simulink model "Attitude_Determination_Iterated"  (R2016b)
settings: Solver=FixedStepDiscrete  StartTime=0.0  StopTime=1  FixedStep=0.1  RelTol=1e-3
undefined symbols (not defined in the file or in its folder): km, s
libraries: dspmathops x4, aerolibtransform2 x1, aerolibgravity2 x1, aerolibcelestial x1
settings Model: Creator=Patipan  LastModifiedBy=Patipan

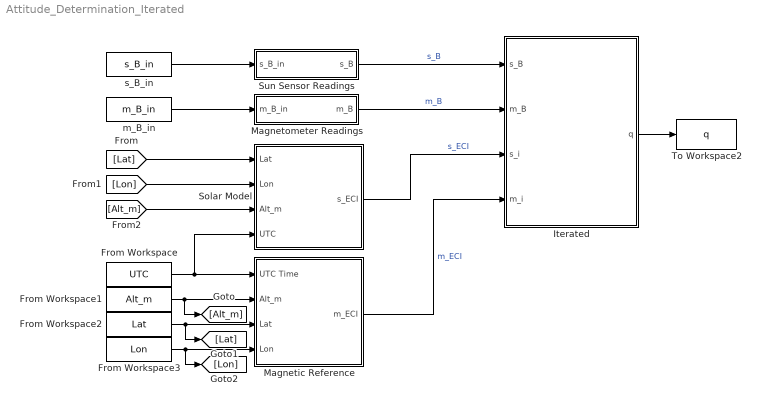
== system Attitude_Determination_Iterated ==
  From Workspace : FromWorkspace  VariableName=UTC  SampleTime=0
  From Workspace1 : FromWorkspace  VariableName=Alt_m  SampleTime=0
  From Workspace2 : FromWorkspace  VariableName=Lat  SampleTime=0
  From Workspace3 : FromWorkspace  VariableName=Lon  SampleTime=0
  Iterated : MATLAB Function  TreatAsAtomicUnit=on
  Magnetic Reference : Subsystem
  Magnetometer Readings : Subsystem
  Solar Model : Subsystem
  Sun Sensor Readings : Subsystem
  To Workspace2 : ToWorkspace  VariableName=q  SampleTime=-1
      settings: Save2DSignal=2-D array (concatenate along first dimension)
  m_B_in : FromWorkspace  VariableName=m_B_in  SampleTime=0
  "s_B_in " : FromWorkspace  VariableName=s_B_in  SampleTime=0
  wires:
  Sun Sensor Readings/1(s_B) -> Iterated/1(s_B)  "s_B"
  Magnetometer Readings/1(m_B) -> Iterated/2(m_B)  "m_B"
  Solar Model/1(s_ECI) -> Iterated/3(s_i)  "s_ECI"
  Magnetic Reference/1(m_ECI) -> Iterated/4(m_i)  "m_ECI"
  "s_B_in "/1 -> Sun Sensor Readings/1(s_B_in)
  m_B_in/1 -> Magnetometer Readings/1(m_B_in)
  From Workspace/1 -> Solar Model/4(UTC), Magnetic Reference/1(UTC Time)
  From Workspace1/1 -> [Alt_m], Magnetic Reference/2(Alt_m)
  From Workspace2/1 -> [Lat], Magnetic Reference/3(Lat)
  From Workspace3/1 -> [Lon], Magnetic Reference/4(Lon)
  [Lat] -> Solar Model/1(Lat)
  [Lon] -> Solar Model/2(Lon)
  [Alt_m] -> Solar Model/3(Alt_m)
  Iterated/1(q) -> To Workspace2/1

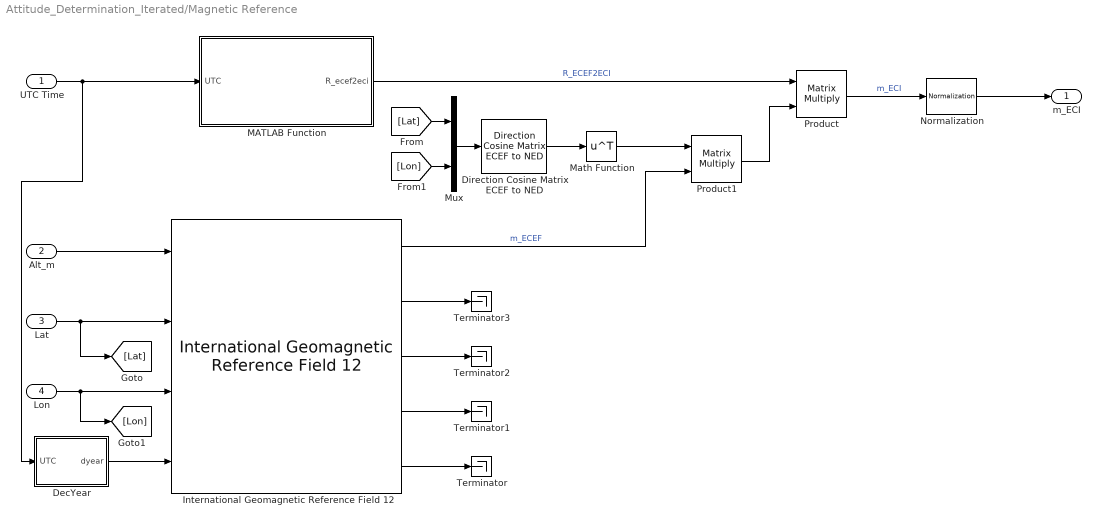
== system Attitude_Determination_Iterated/Magnetic Reference ==
  UTC Time : Inport
  Alt_m : Inport  Port=2
  Lat : Inport  Port=3
  Lon : Inport  Port=4
  DecYear : MATLAB Function  TreatAsAtomicUnit=on
  Direction Cosine Matrix ECEF to NED : aerolibtransform2/Direction Cosine Matrix ECEF to NED
  International Geomagnetic Reference Field 12 : aerolibgravity2/International Geomagnetic Reference Field 12  units=Metric (MKS)  time_in=on  month=January  day=1  year=2020  action=None  sv_out=off
  MATLAB Function : MATLAB Function  TreatAsAtomicUnit=on
  Math Function : Math  Operator=transpose  SaturateOnIntegerOverflow=on
  Mux : Mux  Inputs=2
  Normalization : dspmathops/Normalization  NormType=2-norm  Bias=1e-10  NormOver=Each column  Dimension=1  outputDataTypeStr=Inherit: Same as product output  outputLastDataTypeStr=Inherit: Same as product output  outputMin=[]  outputMax=[]  accumDataTypeStr=Inherit: Same as product output  accumLastDataTypeStr=Inherit: Same as product output  roundingMode=Floor  overflowMode=off
  Product : Product  Multiplication=Matrix(*)
  Product1 : Product  Multiplication=Matrix(*)
  Terminator{,1..3} (4 alike) : Terminator
  m_ECI : Outport
  wires:
  International Geomagnetic Reference Field 12/2 -> Terminator3/1
  International Geomagnetic Reference Field 12/3 -> Terminator2/1
  MATLAB Function/1(R_ecef2eci) -> Product/1  "R_ECEF2ECI"
  Product/1 -> Normalization/1  "m_ECI"
  International Geomagnetic Reference Field 12/4 -> Terminator1/1
  International Geomagnetic Reference Field 12/5 -> Terminator/1
  Lon/1 -> [Lon], International Geomagnetic Reference Field 12/3
  UTC Time/1 -> DecYear/1(UTC), MATLAB Function/1(UTC)
  Alt_m/1 -> International Geomagnetic Reference Field 12/1
  Lat/1 -> [Lat], International Geomagnetic Reference Field 12/2
  DecYear/1(dyear) -> International Geomagnetic Reference Field 12/4
  Mux/1 -> Direction Cosine Matrix ECEF to NED/1
  [Lat] -> Mux/1
  [Lon] -> Mux/2
  International Geomagnetic Reference Field 12/1 -> Product1/2  "m_ECEF"
  Direction Cosine Matrix ECEF to NED/1 -> Math Function/1
  Math Function/1 -> Product1/1
  Product1/1 -> Product/2
  Normalization/1 -> m_ECI/1

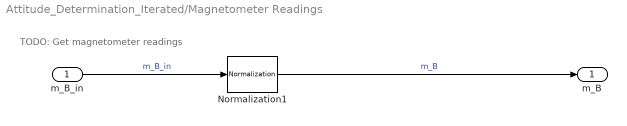
== system Attitude_Determination_Iterated/Magnetometer Readings ==
  note: TODO: Get magnetometer readings
  m_B_in : Inport
  Normalization1 : dspmathops/Normalization  NormType=2-norm  Bias=1e-10  NormOver=Each column  Dimension=1  outputDataTypeStr=Inherit: Same as product output  outputLastDataTypeStr=Inherit: Same as product output  outputMin=[]  outputMax=[]  accumDataTypeStr=Inherit: Same as product output  accumLastDataTypeStr=Inherit: Same as product output  roundingMode=Floor  overflowMode=off
  m_B : Outport
  wires:
  Normalization1/1 -> m_B/1  "m_B"
  m_B_in/1 -> Normalization1/1  "m_B_in"

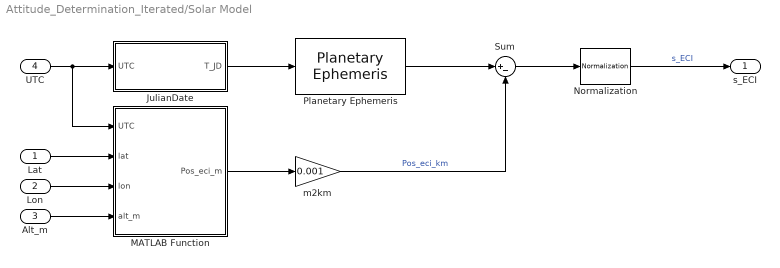
== system Attitude_Determination_Iterated/Solar Model ==
  Lat : Inport
  Lon : Inport  Port=2
  Alt_m : Inport  Port=3
  UTC : Inport  Port=4
  JulianDate : MATLAB Function  TreatAsAtomicUnit=on
  MATLAB Function : MATLAB Function  TreatAsAtomicUnit=on
  Normalization : dspmathops/Normalization  NormType=2-norm  Bias=1e-10  NormOver=Each column  Dimension=1  outputDataTypeStr=Inherit: Same as product output  outputLastDataTypeStr=Inherit: Same as product output  outputMin=[]  outputMax=[]  accumDataTypeStr=Inherit: Same as product output  accumLastDataTypeStr=Inherit: Same as product output  roundingMode=Floor  overflowMode=off
  Planetary Ephemeris : aerolibcelestial/Planetary Ephemeris  kmflag=km,km/s  epochflag=Julian date  de=DE423  nCenter=Earth  nTarget=Sun  errorflag=Error  velflag=off
  Sum : Sum  Inputs=|+-
  m2km : Gain  Gain=0.001
  s_ECI : Outport
  wires:
  Normalization/1 -> s_ECI/1  "s_ECI"
  JulianDate/1(T_JD) -> Planetary Ephemeris/1
  UTC/1 -> MATLAB Function/1(UTC), JulianDate/1(UTC)
  Lat/1 -> MATLAB Function/2(lat)
  Lon/1 -> MATLAB Function/3(lon)
  Alt_m/1 -> MATLAB Function/4(alt_m)
  MATLAB Function/1(Pos_eci_m) -> m2km/1
  Planetary Ephemeris/1 -> Sum/1
  m2km/1 -> Sum/2  "Pos_eci_km"
  Sum/1 -> Normalization/1

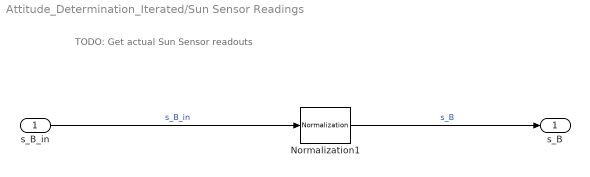
== system Attitude_Determination_Iterated/Sun Sensor Readings ==
  note: TODO: Get actual Sun Sensor readouts
  s_B_in : Inport
  Normalization1 : dspmathops/Normalization  NormType=2-norm  Bias=1e-10  NormOver=Each column  Dimension=1  outputDataTypeStr=Inherit: Same as product output  outputLastDataTypeStr=Inherit: Same as product output  outputMin=[]  outputMax=[]  accumDataTypeStr=Inherit: Same as product output  accumLastDataTypeStr=Inherit: Same as product output  roundingMode=Floor  overflowMode=off
  s_B : Outport
  wires:
  Normalization1/1 -> s_B/1  "s_B"
  s_B_in/1 -> Normalization1/1  "s_B_in"

== matlab function Attitude_Determination_Iterated/Magnetic Reference/MATLAB Function ==
  data: UTC input; R_ecef2eci output
function R_ecef2eci  = ecef2eci(UTC)
% Output rotation matrix from Earth-Centered Earth-Fixed frame to Earth
% Inertial frame from UTC time array.
%  

coder.extrinsic('dcmeci2ecef')

R_eci2ecef = zeros(3, 3);
R_eci2ecef = dcmeci2ecef('IAU-76/FK5', UTC');

R_ecef2eci = R_eci2ecef';
end

== matlab function Attitude_Determination_Iterated/Solar Model/JulianDate ==
  data: UTC input; T_JD output
function T_JD = JulianDate(UTC)

coder.extrinsic('juliandate')
T_JD = 0;
T_JD = juliandate(UTC');

== matlab function Attitude_Determination_Iterated/Magnetic Reference/DecYear ==
  data: UTC input; dyear output
function dyear = DecYear(UTC)

coder.extrinsic('decyear');
dyear = 0;
dyear = decyear(UTC');

== matlab function Attitude_Determination_Iterated/Solar Model/MATLAB Function ==
  data: UTC input; Pos_eci_m output; lat input; lon input; alt_m input
function Pos_eci_m  = lla2eci(UTC, lat, lon, alt_m)
% Output rotation matrix from Earth-Centered Earth-Fixed frame to Earth
% Inertial frame from UTC time array.
%  

coder.extrinsic('lla2eci')

Pos_eci_m = zeros(3, 1);
Pos_eci_m = lla2eci([lat lon alt_m], UTC');

end

== matlab function Attitude_Determination_Iterated/Iterated ==
  data: s_B input; m_B input; s_i input; m_i input; q output
function q  = Iterated(s_B, m_B, s_i, m_i)
% This function is the extended kalman filter for CubeSat attitude
% determination.
% INPUT:
% s_B       Sun vector in body frame from sun sensors
% m_B       Magnetic field vector in body frame from magnetometers
% s_i       Sun vector in inertial frame from planetary ephemeris model
% m_i       Magnetic field vector in inertial frame from IGRF model
%
% OUTPUT:  
% q         Attitude quaternion estimate of the satellite
%

coder.extrinsic('quatrotate');
dt = 0.1; % period for data processing
%% Initialize attitude and error
q = [1 0 0 0];
qprev = [1 0 0 0];
m_est = zeros(3, 1);
s_est = zeros(3, 1);
%% Iterate
for i=1:20
    m_est = quatrotate(q, m_i')';
    s_est = quatrotate(q, s_i')';
    dm = m_B - m_est;
    ds = s_B - s_est;
    
    H = -2*[0               m_est(3)      -m_est(2); 
            -m_est(3)       0             m_est(1);
            m_est(2)        -m_est(1)     0;
            0               s_est(3)      -s_est(2);
            -s_est(3)       0             s_est(1);
            s_est(2)        -s_est(1)     0]; % [6x3] matrix
        
    qe = H\[dm; ds];
    q = quatmultiply(q, [1 qe']);
    q = quatnormalize(q);
    if q(1) < 0
        q = -q;
    end
    qerr = quatmultiply(q, quatconj(qprev));
    if  abs(abs(qerr(1))-1) < 10e-6
        break
    end
    qprev = q;
end
